simulink model "blockdemo"  (Simulink 7.0)
settings: Solver=VariableStepDiscrete  StartTime=0  StopTime=128  MaxStep=1  RelTol=1e-3
InitFcn:
  | %% DSPBuilder Start
  | alt_dspbuilder_update_model(bdroot)
  | %% DSPBuilder End
libraries: allblocks_alteradspbuilder2 x5
settings Model: Creator=mjervis  LastModifiedBy=delphick
settings OptimizationCC: BlockReduction=off  BooleanDataType=off  InlineInvariantSignals=on
settings DebuggingCC: SaveWithParameterizedLinksMsg=none  SignalResolutionControl=TryResolveAllWithWarning  SolverPrmCheckMsg=none  MultiTaskDSMMsg=warning  MultiTaskCondExecSysMsg=none
settings HardwareCC: TargetUnknown=on
settings RTWCC: IncludeERTFirstTime=on
settings GRTTargetCC: TargetFcnLib=ansi_tfl_tmw.mat

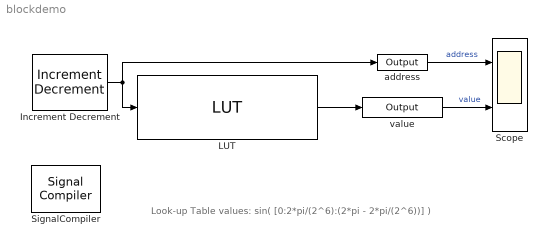
== system blockdemo ==
  note: Look-up Table values: sin( [0:2*pi/(2^6):(2*pi - 2*pi/(2^6))] )
  Increment Decrement : allblocks_alteradspbuilder2/Increment Decrement  BusType=Unsigned Integer  bwl=6  bwr=0  SpecifyClock=off  clr_value=0  direction=Increment  phase_selection=1  use_ena=off  use_sclr=off  pipeline_display=1
  LUT : allblocks_alteradspbuilder2/LUT  addr_width=6  BusType=Signed Fractional  bwl=2  bwr=64  init_array=sin( [0:2*pi/(2^6):(2*pi - 2*pi/(2^6))] )  allowFloatingPointOverride=on  logOutputs=off  logFile=C:\perforce_workspace81\main\dsp_builder2\Documentation\DesignExamples\Tutorials\UnitBlocks\Storage\LUT\tb_blockdemo\blockdemo_LUT.fixedpointlog  use_ena=off  reg_data=on  use_lpm=on  reg_addr=on  ram_type=AUTO  pipeline_display=2
  Scope : Scope  NumInputPorts=2
      settings: YMin=-10~-1.2  YMax=70~1.2
  SignalCompiler : allblocks_alteradspbuilder2/Signal Compiler  DeviceFamily=Stratix IV  DeviceName=AUTO  EnableSignalTap=off  SignalTapDepth=128  UseBoardBlock=off  StpUseDefaultClock=on  StpClock=Clock  ExportDir=C:\Documents and Settings\delphick\My Documents\MATLAB
  address : allblocks_alteradspbuilder2/Output  iofile=C:\perforce_workspace81\main\dsp_builder2\Documentation\DesignExamples\Tutorials\UnitBlocks\Storage\LUT\tb_blockdemo\blockdemo_address.capture  BusType=Unsigned Integer  bwl=8  bwr=0  externalType=Inferred  PORTTYPE=Output  allowFloatingPointOverride=on  logOutputs=off
  value : allblocks_alteradspbuilder2/Output  iofile=C:\perforce_workspace81\main\dsp_builder2\Documentation\DesignExamples\Tutorials\UnitBlocks\Storage\LUT\tb_blockdemo\blockdemo_value.capture  BusType=Signed Fractional  bwl=2  bwr=64  externalType=Inferred  PORTTYPE=Output  allowFloatingPointOverride=on  logOutputs=off
  wires:
  Increment Decrement/1 -> address/1, LUT/1
  LUT/1 -> value/1
  address/1 -> Scope/1  "address"
  value/1 -> Scope/2  "value"
